simulink model "pwm"  (Simulink 7.1)
settings: Solver=ode5  StartTime=0.0  StopTime=5e-3  FixedStep=1e-6  MaxStep=0.000001  RelTol=1e-3
undefined symbols (not defined in the file): amplitude, duty_cycle, on_time, pwm_periode, resolution
libraries: simulink x1
settings Model: Creator=dep19025415  LastModifiedBy=dep19025415

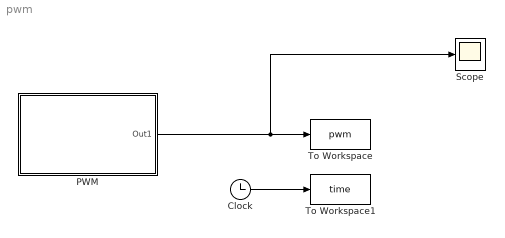
== system pwm ==
  Clock : Clock
      settings: Decimation=10
  PWM : Subsystem  mask{ontime=on_time, amp=amplitude, duty=duty_cycle, tpwm=pwm_periode, max=resolution}
      mask prompts: ontime "On time (s)"; amp "Amplitude (V)"; duty "Duty cycle (%)"; tpwm "PWM period (s)"; max "Resolution"
  Scope : Scope
  To Workspace : ToWorkspace  VariableName=pwm  SampleTime=-1  SaveFormat=Structure
  To Workspace1 : ToWorkspace  VariableName=time  SampleTime=-1  SaveFormat=Structure
  wires:
  PWM/1(Out1) -> To Workspace/1, Scope/1
  Clock/1 -> To Workspace1/1

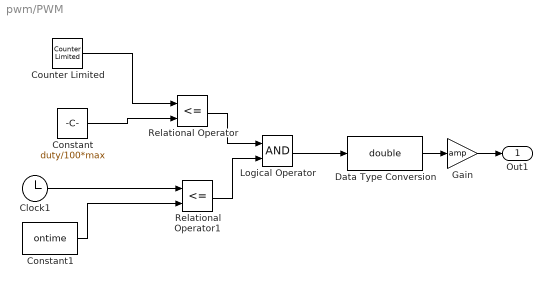
== system pwm/PWM ==
  Clock1 : Clock
      settings: Decimation=10
  Constant : Constant  Value=duty/100*max  OutDataType=sfix(16)  OutScaling=2^0
  Constant1 : Constant  Value=ontime  OutDataType=sfix(16)  OutScaling=2^0
  Counter Limited : simulink/Sources/Counter Limited  SystemSampleTime=-1  uplimit=max  tsamp=tpwm/max
  Data Type Conversion : DataTypeConversion  OutDataTypeMode=double  OutDataType=sfix(16)  OutScaling=2^0  OutDataTypeStr=double
  Gain : Gain  Gain=amp  ParameterDataType=sfix(16)  ParameterScaling=2^0  OutDataType=sfix(16)  OutScaling=2^0
  Logical Operator : Logic  AllPortsSameDT=off  OutDataTypeMode=boolean  OutDataTypeStr=boolean
  Relational Operator : RelationalOperator  Operator=<=  LogicOutDataTypeMode=boolean  OutDataTypeStr=boolean
  Relational Operator1 : RelationalOperator  Operator=<=  LogicOutDataTypeMode=boolean  OutDataTypeStr=boolean
  Out1 : Outport
  wires:
  Counter Limited/1 -> Relational Operator/1
  Constant/1 -> Relational Operator/2
  Clock1/1 -> Relational Operator1/1
  Constant1/1 -> Relational Operator1/2
  Relational Operator/1 -> Logical Operator/1
  Relational Operator1/1 -> Logical Operator/2
  Logical Operator/1 -> Data Type Conversion/1
  Data Type Conversion/1 -> Gain/1
  Gain/1 -> Out1/1
